simulink model "Part9step_realtime"  (R2024b)
settings: Solver=ode3  StartTime=0.0  StopTime=5  FixedStep=0.001  RelTol=1e-3
values from neighbouring files (symbols this model uses):
  Ae = [Arho, zeros(size(Arho, 1), size(A, 1)); B*Crho, A]    [DesignPart9Sine.m]    (also in DesignPart9Step.m = [     Arho, zeros(size(Arho, 1), size(A, 1));      B*Crho, A; Init.m = [0  ,C; zeros(2, 1), A ]; State_space_1324.m = [0  ,C; zeros(2, 1), A ])
  Be = [zeros(size(Arho, 1), 1); B]    [DesignPart9Sine.m]    (also in DesignPart9Step.m; Init.m = [0 ; B]; State_space_1324.m = [0 ; B])
  C = [1, 0]    [DesignPart567.m]    (also in DesignPart8.m; DesignPart9Sine.m; DesignPart9Step.m; Init.m)
  Ce = [zeros(1, size(Arho, 1)), C]    [DesignPart9Sine.m]    (also in DesignPart9Step.m; Init.m = [0 C]; State_space_1324.m = [0 C])
  Cw1 = deg2rad * 1    [DesignPart9Step.m]
  Cw2 = deg2rad * 40    [DesignPart9Step.m]
  delta_est = 1/sqrt(2)    [DesignPart9Step.m]    (also in Init.m)
  Krho = [Crho, K]    [DesignPart9Sine.m]    (also in DesignPart9Step.m)
  L = real(L)    [DesignPart9Sine.m]    (also in DesignPart9Step.m = place(Ae', Ce', ObsvPoles)')
  wc = 2*pi*50    (= 314.159265359)    [DesignPart9Step.m]    (also in Init.m; State_space_1324.m)
undefined symbols (not defined in the file or in its folder): National_Instruments, PCI, sens
libraries: sldrtlib x3, simulink_extras x1
settings Model: SimulationMode=external  ExtModeTrigDuration=1000001  Creator=galeazzolu  LastModifiedBy=galeazzolu
settings DataIOCC: ReturnWorkspaceOutputs=off
settings HardwareCC: ProdBitPerLong=64  ProdHWDeviceType=Intel->x86-64 (Linux 64)
settings RTWCC: Description=Simulink Desktop Real-Time  SystemTargetFile=sldrt.tlc  TemplateMakefile=sldrt.tmf  RTWCompilerOptimization=on
settings CodeAppCC: MaxIdLength=95
settings SimulinkDesktopRealTimeCC: TargetLibSuffix=_sldrt.a  TargetPreCompLibLocation=C:\Program Files\MATLAB\R2024b\toolbox\sldrt\lib\win64  ParMdlRefBuildCompliant=on

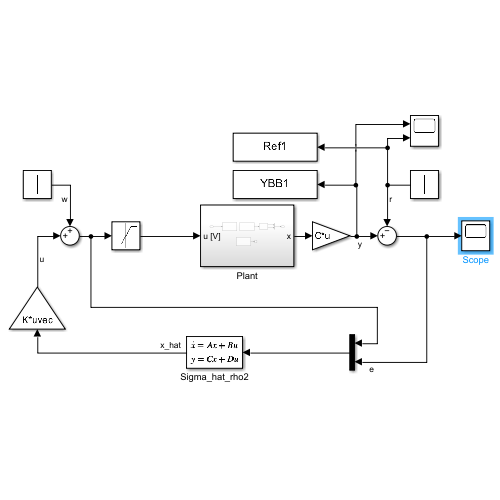
[thumbnail: Simulink's stored preview of the top-level diagram]
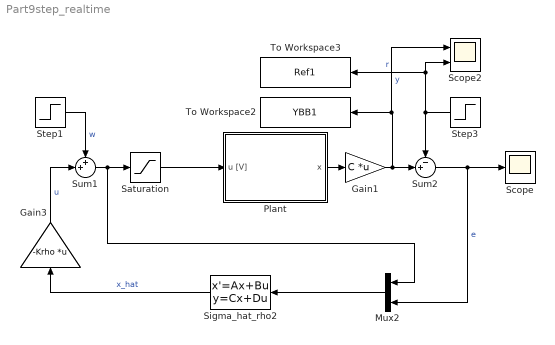
== system Part9step_realtime ==
  Gain1 : Gain  Gain=C  Multiplication=Matrix(K*u)
  Gain3 : Gain  Gain=-Krho  Multiplication=Matrix(K*u) (u vector)
  Mux2 : Mux  Inputs=2
  Plant : Subsystem
  Saturation : Saturate  UpperLimit=10  LowerLimit=-10
  Scope : Scope
  Scope2 : Scope  NumInputPorts=2
  Sigma_hat_rho2 : StateSpace  A=Ae - L*Ce  B=[Be, L]  C=eye(3)  D=zeros(3, 2)  InitialCondition=zeros(3, 1)
  Step1 : Step  After=Cw1  SampleTime=0
  Step3 : Step  After=Cw2  SampleTime=0
  Sum1 : Sum  Inputs=++|
  Sum2 : Sum  Inputs=-+|
  To Workspace2 : ToWorkspace  VariableName=YBB1  SaveFormat=Timeseries  SampleTime=-1
  To Workspace3 : ToWorkspace  VariableName=Ref1  SaveFormat=Timeseries  SampleTime=-1
  wires:
  Sum2/1 -> Scope/1, Mux2/2  "e"
  Plant/1(x) -> Gain1/1
  Sum1/1 -> Mux2/1, Saturation/1
  Sigma_hat_rho2/1 -> Gain3/1  "x_hat"
  Step3/1 -> Sum2/1, Scope2/2, To Workspace3/1  "r"
  Step1/1 -> Sum1/1  "w"
  Gain1/1 -> Scope2/1, To Workspace2/1, Sum2/2  "y"
  Saturation/1 -> Plant/1(u [V])
  Gain3/1 -> Sum1/2  "u"
  Mux2/1 -> Sigma_hat_rho2/1

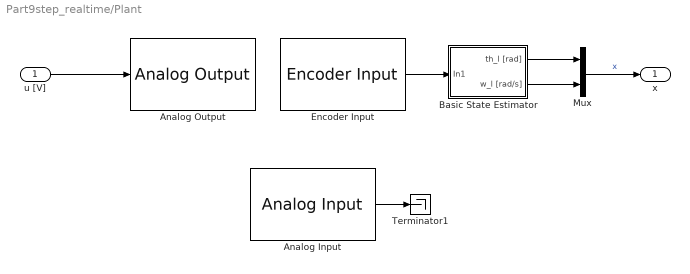
== system Part9step_realtime/Plant ==
  u [V] : Inport
  Analog Input : sldrtlib/Analog Input  SampleTime=-1  MaxMissedTicks=10  ShowMissedTicks=off  YieldWhenWaiting=off  DrvName=National_Instruments/PCI-6221  DrvAddress=4294967295  DrvOptions=[0 0 0 2 0]  Channels=[1,2]  RangeMode=1  VoltRange=1  DataType=1
      settings: AttributesFormatString=National Instruments\nPCI-6221 [auto]
  Analog Output : sldrtlib/Analog Output  SampleTime=-1  MaxMissedTicks=10  ShowMissedTicks=off  YieldWhenWaiting=off  DrvName=National_Instruments/PCI-6221  DrvAddress=4294967295  DrvOptions=[0 0 0 2 0]  Channels=1  RangeMode=1  VoltRange=1  InitialValue=0  FinalValue=0
      settings: AttributesFormatString=National Instruments\nPCI-6221 [auto]
  Basic State Estimator : Subsystem
  Encoder Input : sldrtlib/Encoder Input  SampleTime=-1  MaxMissedTicks=10  ShowMissedTicks=off  YieldWhenWaiting=off  DrvName=National_Instruments/PCI-6221  DrvAddress=4294967295  DrvOptions=[0 0 0 2 0]  Channels=1  QuadMode=3  IndexPulse=1  InputFilter=Inf  DataType=1
      settings: AttributesFormatString=National Instruments\nPCI-6221 [auto]
  Mux : Mux  Inputs=2
  Terminator1 : Terminator
  x : Outport
  wires:
  u [V]/1 -> Analog Output/1
  Encoder Input/1 -> Basic State Estimator/1(In1)
  Mux/1 -> x/1  "x"
  Basic State Estimator/1(th_l [rad]) -> Mux/1
  Basic State Estimator/2(w_l [rad/s]) -> Mux/2
  Analog Input/1 -> Terminator1/1

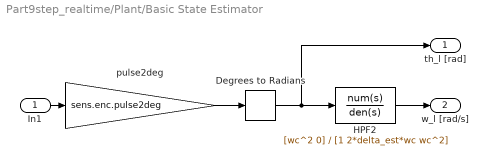
== system Part9step_realtime/Plant/Basic State Estimator ==
  In1 : Inport
  Degrees to Radians : simulink_extras/Transformations/Degrees to Radians
  HPF2 : TransferFcn  Numerator=[wc^2 0]  Denominator=[1 2*delta_est*wc wc^2]
  pulse2deg : Gain  Gain=sens.enc.pulse2deg
  th_l [rad] : Outport
  w_l [rad/s] : Outport  Port=2
  wires:
  pulse2deg/1 -> Degrees to Radians/1
  In1/1 -> pulse2deg/1
  HPF2/1 -> w_l [rad/s]/1
  Degrees to Radians/1 -> th_l [rad]/1, HPF2/1
